simulink model "Three_phase_inverter"  (R2020a)
settings: Solver=VariableStepAuto  StartTime=0.0  StopTime=.06  RelTol=1e-3
libraries: powerlib x15, powerlib_meascontrol x2
settings Model: Creator=User  LastModifiedBy=User

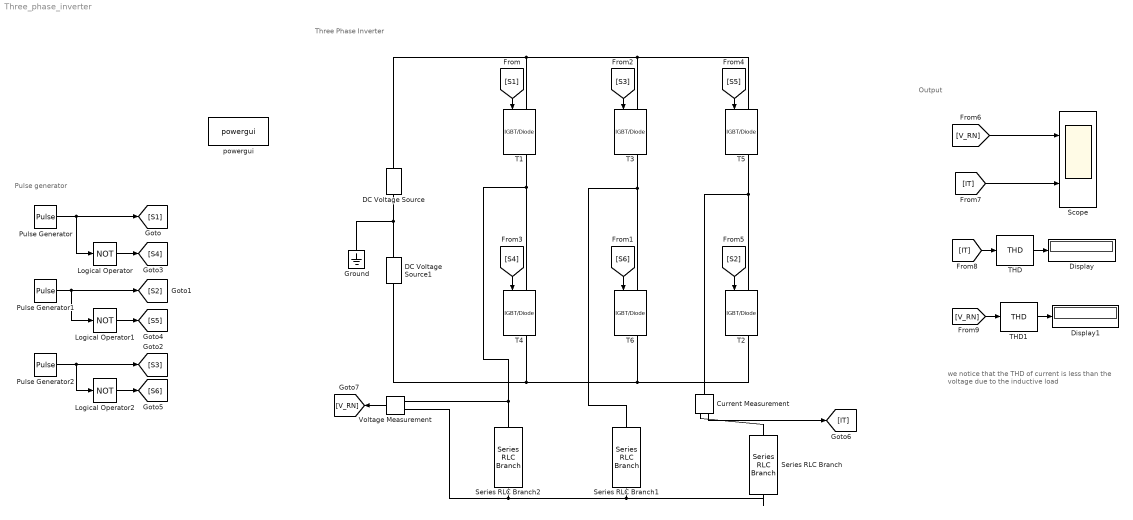
== system Three_phase_inverter ==
  note: Output
  note: we notice that the THD of current is less than the voltage due to the inductive load
  note: Three Phase Inverter
  note: Pulse generator
  Current Measurement : powerlib/Measurements/Current Measurement  PhasorSimulation=off  OutputType=Complex  PSBequivalent=0
  DC Voltage Source : powerlib/Electrical Sources/DC Voltage Source  Amplitude=100  Measurements=None
  DC Voltage Source1 : powerlib/Electrical Sources/DC Voltage Source  Amplitude=100  Measurements=None
  Display : Display
  Display1 : Display
  Ground : powerlib/Elements/Ground  LConnTagsString=a
  Logical Operator : Logic  Operator=NOT  AllPortsSameDT=off  OutDataTypeStr=boolean
  Logical Operator1 : Logic  Operator=NOT  AllPortsSameDT=off  OutDataTypeStr=boolean
  Logical Operator2 : Logic  Operator=NOT  AllPortsSameDT=off  OutDataTypeStr=boolean
  Pulse Generator : DiscretePulseGenerator  PulseType=Time based  Period=.02  PulseWidth=50
  Pulse Generator1 : DiscretePulseGenerator  PulseType=Time based  Period=.02  PulseWidth=50  PhaseDelay=.02*(60/360)
  Pulse Generator2 : DiscretePulseGenerator  PulseType=Time based  Period=.02  PulseWidth=50  PhaseDelay=.02*(120/360)
  Scope : Scope  NumInputPorts=2
  Series RLC Branch : powerlib/Elements/Series RLC Branch  LConnTagsString=__new0  RConnTagsString=__new0  BranchType=RL  Resistance=10  Inductance=50e-3  SetiL0=off  InitialCurrent=0  Capacitance=1e-6  Setx0=off  InitialVoltage=0  Measurements=None
  Series RLC Branch1 : powerlib/Elements/Series RLC Branch  LConnTagsString=__new0  RConnTagsString=__new0  BranchType=RL  Resistance=10  Inductance=50e-3  SetiL0=off  InitialCurrent=0  Capacitance=1e-6  Setx0=off  InitialVoltage=0  Measurements=None
  Series RLC Branch2 : powerlib/Elements/Series RLC Branch  LConnTagsString=__new0  RConnTagsString=__new0  BranchType=RL  Resistance=10  Inductance=50e-3  SetiL0=off  InitialCurrent=0  Capacitance=1e-6  Setx0=off  InitialVoltage=0  Measurements=None
  T{1..6} (6 alike) : powerlib/Power Electronics/IGBT//Diode  Ron=1e-3  Rs=1e5  Cs=inf  Measurements=on
  THD : powerlib_meascontrol/Measurements/THD  Freq=60  Ts=0
  THD1 : powerlib_meascontrol/Measurements/THD  Freq=60  Ts=0
  Voltage Measurement : powerlib/Measurements/Voltage Measurement  PhasorSimulation=off  OutputType=Complex  PSBequivalent=0
  powergui : powerlib/powergui  Priority=1  SimulationMode=Continuous  SampleTime=50e-6  frequency=60  Iterations=50  frequencyindice=0  Pbase=100e6  ErrMax=1e-4  UnitsV=kV  UnitsW=MW  buscounter=0  FunctionMessages=off  echomessages=off  EnableUseOfTLC=off  CurrentSourceSwitches=off  DisableSnubberDevices=on  DisableRonSwitches=on  DisableVfSwitches=on  DisplayEquations=off  AutomaticDiscreteSolvers=off  SolverType=Tustin/Backward Euler (TBE)  Interpol=off  ExternalGateDelay=off  methode=off  Ts=100  x0status=blocks  SPID=on  SwTol=0  HookPort=off  NonlinearTolerance=1e-4  nMaxIteration=100  ContinueOnMaxIteration=off  RestoreLinks=warning  ResistiveCurrentMeasurement=off  Frange=[0:2:500]  Ylog=off  Xlog=on  ShowGrid=off  save=off  variable=ZData  structure=0  ZoomFFT=off  StartTime=0.0  cycles=1  DisplayStyle=1  fundamental=60  FreqAxis=off  MaxFrequency=1000  frequencyindicesteady=1  RmsSteady=1  display=off
  wires:
  Pulse Generator/1 -> [S1], Logical Operator/1
  Pulse Generator1/1 -> [S2], Logical Operator1/1
  [S1] -> T1/1
  [S6] -> T6/1
  [S3] -> T3/1
  [S4] -> T4/1
  Pulse Generator2/1 -> Logical Operator2/1, [S3]
  Logical Operator/1 -> [S4]
  Logical Operator1/1 -> [S5]
  Logical Operator2/1 -> [S6]
  [S5] -> T5/1
  [S2] -> T2/1
  Current Measurement/1 -> [IT]
  Voltage Measurement/1 -> [V_RN]
  [V_RN] -> Scope/1
  [IT] -> Scope/2
  [IT] -> THD/1
  THD/1 -> Display/1
  [V_RN] -> THD1/1
  THD1/1 -> Display1/1
  connections:
  T1/LConn1 -- DC Voltage Source/RConn1 -- T5/LConn1 -- T3/LConn1
  T4/RConn1 -- DC Voltage Source1/LConn1 -- T2/RConn1 -- T6/RConn1
  T1/RConn1 -- Series RLC Branch2/LConn1 -- Voltage Measurement/LConn1 -- T4/LConn1
  DC Voltage Source1/RConn1 -- Ground/LConn1 -- DC Voltage Source/LConn1
  T3/RConn1 -- Series RLC Branch1/LConn1 -- T6/LConn1
  T2/LConn1 -- Current Measurement/LConn1 -- T5/RConn1
  Series RLC Branch/RConn1 -- Voltage Measurement/LConn2 -- Series RLC Branch2/RConn1 -- Series RLC Branch1/RConn1
  Series RLC Branch/LConn1 -- Current Measurement/RConn1
